simulink model "soft_finger_main"  (R2022b)
settings: Solver=VariableStepAuto  StartTime=0.0  StopTime=50  RelTol=1e-3
undefined symbols (not defined in the file): bounds, cf, D, DiscIntNeverNeededParam, Discrete, Fingertip, forceSetPoint, K, M, mylib, rho, sensor_locs, Time, X, Y, Z
libraries: sm_lib x117, nesl_utility x97, fl_lib x81, ee_lib x6, simulink x4, statsLibrary x3, slpidlib x2, deeplib x1, ctrlSharedLib x1
(part 1 of 5)
settings Model: Creator=toby  LastModifiedBy=chapa
settings SolverCC: AlgebraicLoopSolver=TrustRegion
settings DebuggingCC: UnconnectedInputMsg=warning  UnconnectedOutputMsg=warning  UnconnectedLineMsg=warning  SFMachineParentedDataDiag=warning
settings ModelReferenceCC: EnableRefExpFcnMdlSchedulingChecks=on
settings RTWCC: DLArmComputeVersion=19.05
settings ExplorerConfigSet: InternalSimMechanicsExplorerSettings="<ExplorerConfiguration><canonicalview>default</canonicalview><AnimationSetting><BasePlaybackSpeed>1.0</BasePlaybackSpeed><PlaybackSpeedFactor>1.0</PlaybackSpeedFactor></AnimationSetting><TilePanel><TileInfo><Tiles Columns=\"1\" Count=\"1\" Rows=\"1\"><Column Weight=\"1\"/><Row Weight=\"1\"/><Tile Height=\"1\" Width=\"1\" X=\"0\" Y=\"0\"/></Tiles></TileInfo><SceneInfo><SceneViewer><BGColor><R>1</R><G>1</G><B>1</B></BGColor><Camera><DoPerspective>off</DoPerspective><Position><X>0.648695100589207763</X><Y>-0.590632325015253423</Y><Z>0.584680131044784668</Z></Position><Center><X>0.0713448313995819899</X><Y>-0.0132820558256276505</Y><Z>0.0073298618551588552</Z></Center><Up><X>-0.408248290463863073</X><Y>0.408248290463863073</Y><Z>0.816496580927726145</Z></Up><ViewLimDist>1</ViewLimDist><YLim>0.069189024666258106</YLim><XLim>0.106148631121814288</XLim></Camera></SceneViewer></SceneInfo></TilePanel><MechEditorPanel><Cameras/><GfxPanelCameraMap/><VideoCreator><PlaybackSpeedRatio>1.0</PlaybackSpeedRatio><FrameRate>30</FrameRate><VideoFormat>Motion JPEG AVI</VideoFormat><FrameSize>auto</FrameSize></VideoCreator></MechEditorPanel></ExplorerConfiguration>"

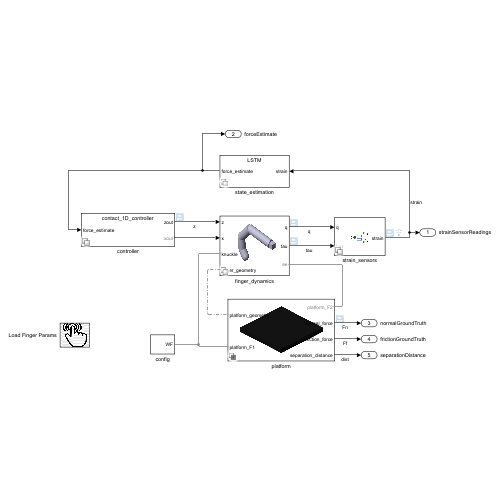
[thumbnail: Simulink's stored preview of the top-level diagram]
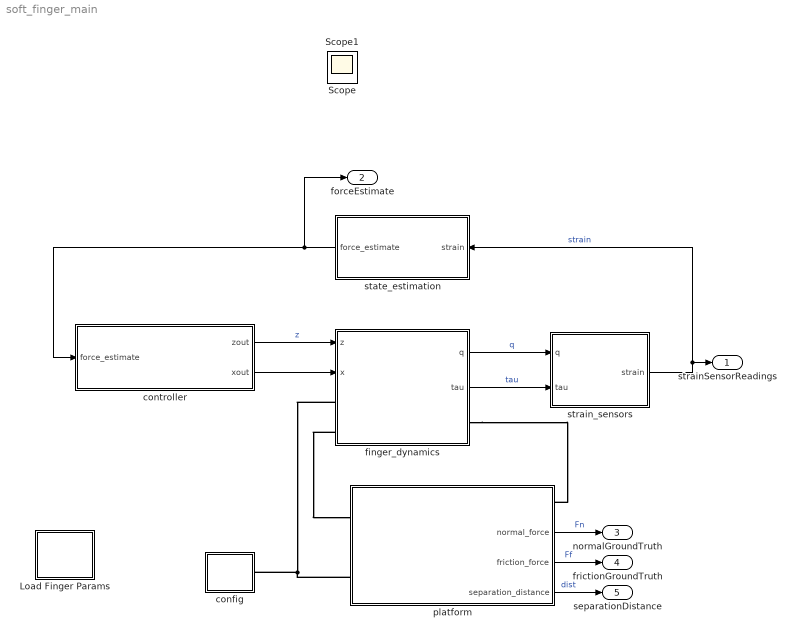
== system soft_finger_main ==
  Load Finger Params : Subsystem
      settings: OpenFcn=loadFingerParams;
      mask Display: image('$imagefile'); % Use "Edit Image" on toolstrip to change.
  config : Subsystem
  controller : Subsystem  Variant=on  VariantControl=Choice
  finger_dynamics : Subsystem  Variant=on  VariantControl=Choice
      mask Display: image('$imagefile'); % Use "Edit Image" on toolstrip to change.
  platform : Subsystem  Variant=on  VariantControlMode=label  VariantControl=Choice  LabelModeActiveChoice=long_2D
      settings: PortSchema="{\"entries\":[{\"content\":{\"sides\":[{\"content\":{\"connectorIds\":[\"LConn1\",\"LConn2\"]},\"type\":\"ConnectorPlacement.EquallySpacedRectSide\",\"uuid\":\"48745db0-03fd-4998-bcf1-1a9aed8c42d1\"},{\"content\":{\"connectorIds\":[\"RConn1\",\"Out1\",\"Out2\",\"Out3\"],\"side\":\"RIGHT\"},\"type\":\"ConnectorPlacement.EquallySpacedRectSide\",\"uuid\":\"a3eff733-8e96-4ac6-b0c1-c9eca8eafbf9\"},{\"content\":{\"connectorIds\":[],\"side\":\"TOP\"},\"type\":\"ConnectorPlacement.EquallySpacedRectSide\",\"uuid\":\"624833be-01c7-4c79-8903-c72d4883aa5d\"}]},\"type\":\"ConnectorPlacement.EquallySpacedConnector\",\"uuid\":\"3e612e1c-fe4d-4d00-a236-ee36b2ab6a58\"}],\"packageUris\":[\"http://schema.mathworks.com/mf0/Connector/R2020b\"],\"version\":\"1.0\"}"
      mask Display: image('$imagefile'); % Use "Edit Image" on toolstrip to change.
  state_estimation : Subsystem  Variant=on  VariantControl=Choice
  strain_sensors : Subsystem  Variant=on  VariantControl=Choice
      mask Display: image('$imagefile'); % Use "Edit Image" on toolstrip to change.
  strainSensorReadings : Outport
  forceEstimate : Outport  Port=2
  normalGroundTruth : Outport  Port=3
  frictionGroundTruth : Outport  Port=4
  separationDistance : Outport  Port=5
  Scope : Scope
  Scope1 : Scope
  wires:
  strain_sensors/1(strain) -> state_estimation/1(strain), strainSensorReadings/1  "strain"
  platform/1(normal_force) -> normalGroundTruth/1  "Fn"
  controller/1(zout) -> finger_dynamics/1(z)  "z"
  finger_dynamics/1(q) -> strain_sensors/1(q)  "q"
  state_estimation/1(force_estimate) -> controller/1(force_estimate), forceEstimate/1
  controller/2(xout) -> finger_dynamics/2(x)
  platform/2(friction_force) -> frictionGroundTruth/1  "Ff"
  platform/3(separation_distance) -> separationDistance/1  "dist"
  finger_dynamics/2(tau) -> strain_sensors/2(tau)  "tau"
  connections:
  platform/LConn2 -- config/RConn1 -- finger_dynamics/LConn1
  finger_dynamics/LConn2 -- platform/LConn1
  finger_dynamics/RConn1 -- platform/RConn1

== system soft_finger_main/Load Finger Params ==

== system soft_finger_main/config ==
  Mechanism Configuration : sm_lib/Utilities/Mechanism Configuration  UniformGravity=Constant  GravityVector=[0 0 -9.80665]  GravityUnits=m/s^2  LinearizationDelta=0.001  JointModeTransitionNonlinearIterations=2
  Solver Configuration : nesl_utility/Solver Configuration  PhysicalDomain=network_engine_domain  SubClassName=solver  LeftPortType=input  RightPortType=generic  Tones=[]  Harmonics=[]  SimulateNoise=off  Profile=off  UseLocalSampling=off  EnableSwitchedLinearOptims=on  FrequencyDomain=off  UseCCode=off  RelTol=0.001  AbsTol=1e-06  MinStep=1e-09  ToWorkspace=off  RevertToSquareIcSolve=off  NumHomotopyIterations=100  PhasorMode=off  PhasorModeNumHarmonics=1  ConsistencySolver=NEWTON_XTOL_AFTER_FTOL  IndexReductionMethod=DerivativeReplacement  DoDC=off  ResidualTolerance=1e-09  ConsistencyTolSource=GLOBAL  ConsistencyAbsTol=0.001  ConsistencyRelTol=0.001  ConsistencyTolFactor=0.001  UseLocalSolver=off  LocalSolverChoice=NE_BACKWARD_EULER_ADVANCER  ResolveIndetEquations=on  FunctionEvalNumThread=1  LocalSolverSampleTime=0.001  DoFixedCost=off  MaxNonlinIter=3  MaxModeIter=2  ComputeImpulses=off  ImpulseIterations=2  LinearAlgebra=auto  LinearAlgebraNumThread=0  EquationFormulation=NE_TIME_EF  DelaysMemoryBudget=1024  AutomaticFiltering=on  FilteringTimeConstant=0.001  PartitionStorageMethod=AS_NEEDED  PartitionMemoryBudget=1024  PartitionMethod=ROBUST
  World Frame : sm_lib/Frames and Transforms/World Frame
  WF : PMIOPort  Side=Right
  connections:
  Mechanism Configuration/RConn1 -- WF/RConn1 -- World Frame/RConn1 -- Solver Configuration/RConn1

== system soft_finger_main/controller ==
  force_estimate : Inport
  contact_1D_controller : Subsystem  VariantControl=controller_choice==1
  contact_2D_controller : Subsystem  VariantControl=controller_choice==2
  custom : Subsystem  VariantControl=controller_choice==2
  random_walker_xz : Subsystem  VariantControl=controller_choice==4
  random_walker_z : Subsystem  VariantControl=controller_choice==3
  zout : Outport
  xout : Outport  Port=2

== system soft_finger_main/finger_dynamics ==
  z : Inport
  x : Inport  Port=2
  XZ Translation at Base : Subsystem  VariantControl=plant_choice == 2
  Z Translation at Base : Subsystem  VariantControl=plant_choice == 1
  knuckle : PMIOPort  Side=Left
  finger_geometry : PMIOPort  Port=2  Side=Left
  ee : PMIOPort  Port=3  Side=Right
  q : Outport
  tau : Outport  Port=2

== system soft_finger_main/platform ==
  long_platform : Subsystem  VariantControl=long_2D
  short_platform : Subsystem  VariantControl=short_1D
  platform_geometry : PMIOPort  Side=Left
  platform_F1 : PMIOPort  Port=2  Side=Left
  platform_F2 : PMIOPort  Port=3  Side=Right
  normal_force : Outport
  friction_force : Outport  Port=2
  separation_distance : Outport  Port=3

== system soft_finger_main/state_estimation ==
  strain : Inport
  LSTM : Subsystem  VariantControl=observer_choice == 3
      settings: AttributesFormatString=(Experimental)
  SVM : Subsystem  VariantControl=observer_choice == 4
  bagged_ensemble : Subsystem  VariantControl=observer_choice == 1
  bagged_ensemble_with_friction : Subsystem  VariantControl=observer_choice == 2
  custom : Subsystem  VariantControl=observer_choice == 8
  kalman_filter : Subsystem  VariantControl=observer_choice == 7
      settings: AttributesFormatString=(Experimental)
  linear_regression : Subsystem  VariantControl=observer_choice == 5
  off : Subsystem  VariantControl=observer_choice == 9
  state_space_observer : Subsystem  VariantControl=observer_choice == 6
      settings: AttributesFormatString=(Experimental)
  force_estimate : Outport

== system soft_finger_main/strain_sensors ==
  q : Inport
  tau : Inport  Port=2
  drifting_strain_sensor : Subsystem  VariantControl=sensor_choice == 1
  ssc_strain_sensor : Subsystem  VariantControl=sensor_choice == 2
  strain : Outport

== system soft_finger_main/controller/contact_1D_controller ==
  note: adjust the force set point and observe at which force the mechanism collapses
  force_estimate : Inport
  Bus Selector : BusSelector  OutputSignals=normal
  Delay2 : Delay  DelayLength=1;  InitialCondition=0;
  PID Controller : slpidlib/PID Controller  Controller=PID  Form=Parallel  TimeDomain=Discrete-time  UseExternalTs=off  SampleTime=-1  IntegratorMethod=Forward Euler  FilterMethod=Forward Euler  ControllerParametersSource=internal  P=1.4  I=0  UseKiTs=off  D=0.05  N=1  UseFilter=on  TunerSelectOption=Frequency Response Based  InitialConditionSource=internal  InitialConditionForIntegrator=0  InitialConditionForFilter=0  DifferentiatorICPrevScaledInput=0  ExternalReset=none  TrackingMode=off  Kt=1  LimitOutput=off  SatLimitsSource=internal  UpperSaturationLimit=inf  LowerSaturationLimit=-inf  LinearizeAsGain=on  AntiWindupMode=none  Kb=1  LimitIntegrator=off  UpperIntegratorSaturationLimit=inf  LowerIntegratorSaturationLimit=-inf  POutMin=[]  POutMax=[]  IOutMin=[]  IOutMax=[]  DOutMin=[]  DOutMax=[]  NOutMin=[]  NOutMax=[]  SumOutMin=[]  SumOutMax=[]  SaturationOutMin=[]  SaturationOutMax=[]  PParamMin=[]  PParamMax=[]  IParamMin=[]  IParamMax=[]  DParamMin=[]  DParamMax=[]  NParamMin=[]  NParamMax=[]  KbParamMin=[]  KbParamMax=[]  KtParamMin=[]  KtParamMax=[]  KbOutMin=[]  KbOutMax=[]  KtOutMin=[]  KtOutMax=[]  IntegratorOutMin=[]  IntegratorOutMax=[]  FilterOutMin=[]  FilterOutMax=[]  SumI1OutMin=[]  SumI1OutMax=[]  SumI2OutMin=[]  SumI2OutMax=[]  SumI3OutMin=[]  SumI3OutMax=[]  SumI4OutMin=[]  SumI4OutMax=[]  SumDOutMin=[]  SumDOutMax=[]  DifferentiatorOutMin=[]  DifferentiatorOutMax=[]  FilterDiffOutCoefMin=[]  FilterDiffOutCoefMax=[]  ReciprocalOutMin=[]  ReciprocalOutMax=[]  SumDenOutMin=[]  SumDenOutMax=[]  SumNumOutMin=[]  SumNumOutMax=[]  DivideOutMin=[]  DivideOutMax=[]  UdiffTsProdOutMin=[]  UdiffTsProdOutMax=[]  NTsProdOutMin=[]  NTsProdOutMax=[]  UintegralTsProdOutMin=[]  UintegralTsProdOutMax=[]  UngainTsProdOutMin=[]  UngainTsProdOutMax=[]  ClampingZeroOutDataTypeStr=Inherit: Inherit via back propagation  ClampingZeroOutMin=[]  ClampingZeroOutMax=[]  FilterDenConstantOutDataTypeStr=Inherit: Inherit via back propagation  FilterDenConstantOutMin=[]  FilterDenConstantOutMax=[]  PCopyOutDataTypeStr=Inherit: Inherit via back propagation  PCopyOutMin=[]  PCopyOutMax=[]  NCopyOutDataTypeStr=Inherit: Inherit via back propagation  NCopyOutMin=[]  NCopyOutMax=[]  IntegratorContinuousStateAttributes=''  IntegratorStateMustResolveToSignalObject=off  IntegratorRTWStateStorageClass=Auto  FilterContinuousStateAttributes=''  FilterStateMustResolveToSignalObject=off  FilterRTWStateStorageClass=Auto  ParallelPVariant=InternalParameters  IdealPVariant=Disabled  IVariant=InternalParameters  DVariant=InternalParameters  IntegratorVariant=Discrete  SatVariant=Disabled  AWVariant=Passthrough  PCopyVariant=Disabled  TRVariant=Disabled  FdbkBlocksVariant=Forward  IdealPFdbkVariant=Disabled  SatFdbkVariant=Disabled  DerivativeFilterVariant=ForwardEulerFilter  NVariant=InternalParameters  NCopyVariant=Disabled  FilterICVariant=InternalICsFilter  IntegratorICVariant=InternalICs  ExternalResetVariant=Disabled  TRSumVariant=Passthrough  SumFdbkVariant=Disabled  SumVariant=Sum_PID  TsampFilterVariant=InternalTs  TsampNgainVariant=Passthrough  TsampIntegralVariant=Passthrough  ExternalSaturationOutDataTypeStr=Inherit: Same as second input
  Sum1 : Sum  Inputs=|+-
  Sum2 : Sum  Inputs=|-+
  Zero-Order Hold : ZeroOrderHold  SampleTime=-1
  acceleration limiter : Subsystem
  desired_force : Constant  Value=forceSetPoint
  zout : Outport
  wires:
  force_estimate/1 -> Bus Selector/1
  Sum1/1 -> PID Controller/1  "forceErr"
  acceleration limiter/1(zout) -> zout/1
  Sum2/1 -> Zero-Order Hold/1, Delay2/1  "pos_next"
  Delay2/1 -> Sum2/2  "pos_now"
  Zero-Order Hold/1 -> acceleration limiter/1(pos_next)
  PID Controller/1 -> Sum2/1  "pos_fb_correction"
  desired_force/1 -> Sum1/1  "sp"
  Bus Selector/1 -> Sum1/2  "<normal>"

== system soft_finger_main/controller/contact_2D_controller ==
  note: adjust the force set point and observe at which force the mechanism collapses
  force_estimate : Inport
  Bus Selector : BusSelector  OutputSignals=normal
  Bus Selector1 : BusSelector  OutputSignals=friction
  Delay2 : Delay  DelayLength=1;  InitialCondition=0;
  PID Controller : slpidlib/PID Controller  Controller=PID  Form=Parallel  TimeDomain=Discrete-time  UseExternalTs=off  SampleTime=-1  IntegratorMethod=Forward Euler  FilterMethod=Forward Euler  ControllerParametersSource=internal  P=1.4  I=0  UseKiTs=off  D=0.05  N=1  UseFilter=on  TunerSelectOption=Frequency Response Based  InitialConditionSource=internal  InitialConditionForIntegrator=0  InitialConditionForFilter=0  DifferentiatorICPrevScaledInput=0  ExternalReset=none  TrackingMode=off  Kt=1  LimitOutput=off  SatLimitsSource=internal  UpperSaturationLimit=inf  LowerSaturationLimit=-inf  LinearizeAsGain=on  AntiWindupMode=none  Kb=1  LimitIntegrator=off  UpperIntegratorSaturationLimit=inf  LowerIntegratorSaturationLimit=-inf  POutMin=[]  POutMax=[]  IOutMin=[]  IOutMax=[]  DOutMin=[]  DOutMax=[]  NOutMin=[]  NOutMax=[]  SumOutMin=[]  SumOutMax=[]  SaturationOutMin=[]  SaturationOutMax=[]  PParamMin=[]  PParamMax=[]  IParamMin=[]  IParamMax=[]  DParamMin=[]  DParamMax=[]  NParamMin=[]  NParamMax=[]  KbParamMin=[]  KbParamMax=[]  KtParamMin=[]  KtParamMax=[]  KbOutMin=[]  KbOutMax=[]  KtOutMin=[]  KtOutMax=[]  IntegratorOutMin=[]  IntegratorOutMax=[]  FilterOutMin=[]  FilterOutMax=[]  SumI1OutMin=[]  SumI1OutMax=[]  SumI2OutMin=[]  SumI2OutMax=[]  SumI3OutMin=[]  SumI3OutMax=[]  SumI4OutMin=[]  SumI4OutMax=[]  SumDOutMin=[]  SumDOutMax=[]  DifferentiatorOutMin=[]  DifferentiatorOutMax=[]  FilterDiffOutCoefMin=[]  FilterDiffOutCoefMax=[]  ReciprocalOutMin=[]  ReciprocalOutMax=[]  SumDenOutMin=[]  SumDenOutMax=[]  SumNumOutMin=[]  SumNumOutMax=[]  DivideOutMin=[]  DivideOutMax=[]  UdiffTsProdOutMin=[]  UdiffTsProdOutMax=[]  NTsProdOutMin=[]  NTsProdOutMax=[]  UintegralTsProdOutMin=[]  UintegralTsProdOutMax=[]  UngainTsProdOutMin=[]  UngainTsProdOutMax=[]  ClampingZeroOutDataTypeStr=Inherit: Inherit via back propagation  ClampingZeroOutMin=[]  ClampingZeroOutMax=[]  FilterDenConstantOutDataTypeStr=Inherit: Inherit via back propagation  FilterDenConstantOutMin=[]  FilterDenConstantOutMax=[]  PCopyOutDataTypeStr=Inherit: Inherit via back propagation  PCopyOutMin=[]  PCopyOutMax=[]  NCopyOutDataTypeStr=Inherit: Inherit via back propagation  NCopyOutMin=[]  NCopyOutMax=[]  IntegratorContinuousStateAttributes=''  IntegratorStateMustResolveToSignalObject=off  IntegratorRTWStateStorageClass=Auto  FilterContinuousStateAttributes=''  FilterStateMustResolveToSignalObject=off  FilterRTWStateStorageClass=Auto  ParallelPVariant=InternalParameters  IdealPVariant=Disabled  IVariant=InternalParameters  DVariant=InternalParameters  IntegratorVariant=Discrete  SatVariant=Disabled  AWVariant=Passthrough  PCopyVariant=Disabled  TRVariant=Disabled  FdbkBlocksVariant=Forward  IdealPFdbkVariant=Disabled  SatFdbkVariant=Disabled  DerivativeFilterVariant=ForwardEulerFilter  NVariant=InternalParameters  NCopyVariant=Disabled  FilterICVariant=InternalICsFilter  IntegratorICVariant=InternalICs  ExternalResetVariant=Disabled  TRSumVariant=Passthrough  SumFdbkVariant=Disabled  SumVariant=Sum_PID  TsampFilterVariant=InternalTs  TsampNgainVariant=Passthrough  TsampIntegralVariant=Passthrough  ExternalSaturationOutDataTypeStr=Inherit: Same as second input
  Sine Wave : Sin  Amplitude=5  Frequency=0.5  SampleTime=0
  Sum1 : Sum  Inputs=|+-
  Sum2 : Sum  Inputs=|-+
  Terminator : Terminator
  Zero-Order Hold : ZeroOrderHold  SampleTime=-1
  acceleration limiter : Subsystem
  desired_force : Constant  Value=0.1
  zout : Outport
  xout : Outport  Port=2
  wires:
  PID Controller/1 -> Sum2/1  "pos_fb_correction"
  Zero-Order Hold/1 -> acceleration limiter/1(pos_next)
  Delay2/1 -> Sum2/2  "pos_now"
  Sum2/1 -> Delay2/1, Zero-Order Hold/1  "pos_next"
  acceleration limiter/1(zout) -> zout/1
  Sum1/1 -> PID Controller/1  "forceErr"
  Sine Wave/1 -> xout/1  "xref"
  desired_force/1 -> Sum1/1  "sp"
  force_estimate/1 -> Bus Selector1/1, Bus Selector/1
  Bus Selector/1 -> Sum1/2  "<normal>"
  Bus Selector1/1 -> Terminator/1  "<friction>"

== system soft_finger_main/controller/custom ==
  force_estimate : Inport
  Bus Selector : BusSelector  OutputSignals=normal
  Bus Selector1 : BusSelector  OutputSignals=friction
  Constant : Constant  Value=0
  Constant1 : Constant  Value=0
  Terminator : Terminator
  Terminator1 : Terminator
  zout : Outport
  xout : Outport  Port=2
  wires:
  Bus Selector1/1 -> Terminator/1  "<friction>"
  force_estimate/1 -> Bus Selector/1, Bus Selector1/1
  Bus Selector/1 -> Terminator1/1  "<normal>"
  Constant/1 -> zout/1
  Constant1/1 -> xout/1

== system soft_finger_main/controller/random_walker_xz ==
  Add1 : Sum  Inputs=+-+
  Add2 : Sum  Inputs=+-+
  Saturation : Saturate  UpperLimit=bounds(1)  LowerLimit=bounds(2)
  Saturation1 : Saturate  UpperLimit=10  LowerLimit=-10
  Sum : Sum  Inputs=-+|
  Sum1 : Sum  Inputs=-+|
  Unit Delay{1..4} (4 alike) : UnitDelay  SampleTime=-1  HasFrameUpgradeWarning=on
  random dx : RandomNumber  Variance=10  SampleTime=0.1
  random dz : RandomNumber  Variance=0.1  Seed=1  SampleTime=0.1
  zout : Outport
  xout : Outport  Port=2
  wires:
  Unit Delay1/1 -> Add1/3  "ztminus1"
  random dz/1 -> Add1/1
  Add1/1 -> Sum/2, Saturation/1, Unit Delay1/1  "zt"
  Sum/1 -> Unit Delay3/1  "anitwindupz"
  Saturation/1 -> Sum/1, zout/1  "zout"
  Saturation1/1 -> xout/1, Sum1/1  "xout"
  Sum1/1 -> Unit Delay4/1  "anitwindupx"
  Add2/1 -> Saturation1/1, Sum1/2, Unit Delay2/1  "xt"
  random dx/1 -> Add2/1
  Unit Delay2/1 -> Add2/3  "xtminus1"
  Unit Delay3/1 -> Add1/2  "ztminus1"
  Unit Delay4/1 -> Add2/2  "ztminus1"

== system soft_finger_main/controller/random_walker_z ==
  Add1 : Sum  Inputs=+-+
  Constant6 : Constant  Commented=on  Value=[bounds]
  Constant7 : Constant  Commented=on  Value=cf
  Delay : Delay  Commented=on  DelayLength=1;  InitialCondition=[10, 0, 1, 1, 1];
  Demux : Demux  Commented=on  Outputs=5
  MATLAB Function2 : MATLAB Function  Commented=on  TreatAsAtomicUnit=on
  Mux1 : Mux  Commented=on  Inputs=5
  Rate Transition : RateTransition  Commented=on  InitialCondition=0;  OutPortSampleTime=1/cf;
  Saturation : Saturate  UpperLimit=bounds(1)  LowerLimit=bounds(2)
  Sum : Sum  Inputs=-+|
  Unit Delay1 : UnitDelay  SampleTime=-1  HasFrameUpgradeWarning=on
  Unit Delay2 : UnitDelay  SampleTime=-1  HasFrameUpgradeWarning=on
  acceleration limiter : Subsystem  Commented=on
  random dz : RandomNumber  Variance=0.1  Seed=1  SampleTime=0.1
  zout : Outport
  wires:
  Delay/1 -> Demux/1
  Demux/5 -> MATLAB Function2/5("step_no ")
  Demux/1 -> MATLAB Function2/1(pos_now)
  MATLAB Function2/2(pos_goal) -> Mux1/2
  Demux/3 -> MATLAB Function2/3("thres ")
  MATLAB Function2/5(step_no) -> Mux1/5
  Demux/4 -> MATLAB Function2/4("batch ")
  Demux/2 -> MATLAB Function2/2("pos_goal ")
  MATLAB Function2/4(batch) -> Mux1/4
  Rate Transition/1 -> Delay/1
  Mux1/1 -> Rate Transition/1
  MATLAB Function2/1(pos_next) -> Mux1/1, acceleration limiter/1(pos_next)
  Constant7/1 -> MATLAB Function2/7(cf)
  Constant6/1 -> MATLAB Function2/6(bounds)
  MATLAB Function2/3(thres) -> Mux1/3
  acceleration limiter/1(zout) -> ?
  Sum/1 -> Unit Delay2/1  "anitwindupz"
  random dz/1 -> Add1/1
  Unit Delay1/1 -> Add1/3  "ztminus1"
  Saturation/1 -> zout/1, Sum/1  "zout"
  Add1/1 -> Sum/2, Saturation/1, Unit Delay1/1  "zt"
  Unit Delay2/1 -> Add1/2  "ztminus1"

== system soft_finger_main/finger_dynamics/XZ Translation at Base ==
  z : Inport
  x : Inport  Port=2
  Terminator : Terminator
  finger : Subsystem
      mask Display: image('$imagefile'); % Use "Edit Image" on toolstrip to change.
  knuckle : PMIOPort  Side=Left
  finger_geometry : PMIOPort  Port=2  Side=Left
  ee : PMIOPort  Port=3  Side=Right
  q : Outport
  tau : Outport  Port=2
  wires:
  finger/1(joint_angles) -> q/1  "q"
  z/1 -> finger/1(z)
  x/1 -> finger/2(x)
  finger/3(joint_torques) -> tau/1
  finger/2(joint_forces) -> Terminator/1
  connections:
  knuckle/RConn1 -- finger/LConn1
  finger/LConn2 -- finger_geometry/RConn1
  finger/RConn1 -- ee/RConn1

== system soft_finger_main/finger_dynamics/Z Translation at Base ==
  z : Inport
  Terminator : Terminator
  finger : Subsystem
      mask Display: image('$imagefile'); % Use "Edit Image" on toolstrip to change.
  knuckle : PMIOPort  Side=Left
  finger_geometry : PMIOPort  Port=2  Side=Left
  ee : PMIOPort  Port=3  Side=Right
  q : Outport
  tau : Outport  Port=2
  wires:
  z/1 -> finger/1(z)
  finger/1(joint_angles) -> q/1  "q"
  finger/3(joint_torques) -> tau/1  "tau"
  finger/2(joint_forces) -> Terminator/1
  connections:
  ee/RConn1 -- finger/RConn1
  finger_geometry/RConn1 -- finger/LConn2
  knuckle/RConn1 -- finger/LConn1

== system soft_finger_main/platform/long_platform ==
  platform : Subsystem
      settings: PortSchema="{\"entries\":[{\"content\":{\"sides\":[{\"content\":{\"connectorIds\":[\"LConn1\",\"LConn2\"]},\"type\":\"ConnectorPlacement.EquallySpacedRectSide\",\"uuid\":\"6339b0d2-d5db-4d9b-bf7c-b55391eb7ced\"},{\"content\":{\"connectorIds\":[\"RConn1\",\"Out1\",\"Out2\",\"Out3\"],\"side\":\"RIGHT\"},\"type\":\"ConnectorPlacement.EquallySpacedRectSide\",\"uuid\":\"c0a265d5-31ed-4e5e-b9ed-737d24bd79ad\"},{\"content\":{\"connectorIds\":[],\"side\":\"TOP\"},\"type\":\"ConnectorPlacement.EquallySpacedRectSide\",\"uuid\":\"95fda260-2475-4278-80fa-e6b57f61896e\"}]},\"type\":\"ConnectorPlacement.EquallySpacedConnector\",\"uuid\":\"d01ea818-4985-47a8-ad3c-f52aaf4b2cf0\"}],\"packageUris\":[\"http://schema.mathworks.com/mf0/Connector/R2020b\"],\"version\":\"1.0\"}"
      mask Display: image('$imagefile'); % Use "Edit Image" on toolstrip to change.
  platform_geometry : PMIOPort  Side=Left
  platform_F1 : PMIOPort  Port=2  Side=Left
  platform_F2 : PMIOPort  Port=3  Side=Right
  normal_force : Outport
  friction_force : Outport  Port=2
  separation_distance : Outport  Port=3
  wires:
  platform/1(normal_force) -> normal_force/1  "nfgt"
  platform/2(friction_force) -> friction_force/1  "ffgt"
  platform/3(separation_distance) -> separation_distance/1  "dist"
  connections:
  platform/LConn2 -- platform_F1/RConn1
  platform/RConn1 -- platform_F2/RConn1
  platform/LConn1 -- platform_geometry/RConn1

== system soft_finger_main/platform/short_platform ==
  platform : Subsystem
      settings: PortSchema="{\"entries\":[{\"content\":{\"sides\":[{\"content\":{\"connectorIds\":[\"LConn1\",\"LConn2\"]},\"type\":\"ConnectorPlacement.EquallySpacedRectSide\",\"uuid\":\"6339b0d2-d5db-4d9b-bf7c-b55391eb7ced\"},{\"content\":{\"connectorIds\":[\"RConn1\",\"Out1\"],\"side\":\"RIGHT\"},\"type\":\"ConnectorPlacement.EquallySpacedRectSide\",\"uuid\":\"c0a265d5-31ed-4e5e-b9ed-737d24bd79ad\"},{\"content\":{\"connectorIds\":[],\"side\":\"TOP\"},\"type\":\"ConnectorPlacement.EquallySpacedRectSide\",\"uuid\":\"95fda260-2475-4278-80fa-e6b57f61896e\"}]},\"type\":\"ConnectorPlacement.EquallySpacedConnector\",\"uuid\":\"d01ea818-4985-47a8-ad3c-f52aaf4b2cf0\"}],\"packageUris\":[\"http://schema.mathworks.com/mf0/Connector/R2020b\"],\"version\":\"1.0\"}"
      mask Display: image('$imagefile'); % Use "Edit Image" on toolstrip to change.
  platform_geometry : PMIOPort  Side=Left
  platform_F1 : PMIOPort  Port=2  Side=Left
  platform_F2 : PMIOPort  Port=3  Side=Right
  normal_force : Outport
  wires:
  platform/1(normal_force) -> normal_force/1
  connections:
  platform/LConn1 -- platform_geometry/RConn1
  platform/RConn1 -- platform_F2/RConn1
  platform_F1/RConn1 -- platform/LConn2

== system soft_finger_main/state_estimation/LSTM ==
  strain : Inport
  Bus Creator : BusCreator  Inputs=1
  Rate Transition : RateTransition  InitialCondition=0;  OutPortSampleTime=1/cf;
  Stateful Predict : deeplib/Stateful Predict  Network=Network from MAT-file  NetworkFunction=untitled  NetworkFilePath=ml_models\lstm2.mat  InputDataFormats={ '', '' }  SampleTime=0.04  ForceInterpretedSim=off  EnableDLNetwork=on
  Unit Delay : UnitDelay  SampleTime=-1  HasFrameUpgradeWarning=on
  force_estimate : Outport
  wires:
  strain/1 -> Unit Delay/1
  Stateful Predict/1 -> Rate Transition/1
  Unit Delay/1 -> Stateful Predict/1
  Rate Transition/1 -> Bus Creator/1  "normal"
  Bus Creator/1 -> force_estimate/1

== system soft_finger_main/state_estimation/SVM ==
  strain : Inport
  Bus Creator : BusCreator  Inputs=1
  MATLAB Function : MATLAB Function  TreatAsAtomicUnit=on
  Rate Transition : RateTransition  InitialCondition=0;  OutPortSampleTime=1/cf;
  Transpose : Math  Operator=transpose
  Unit Delay : UnitDelay  SampleTime=-1  HasFrameUpgradeWarning=on
  force_estimate : Outport
  wires:
  Unit Delay/1 -> Transpose/1
  MATLAB Function/1(force) -> Rate Transition/1
  strain/1 -> Unit Delay/1
  Transpose/1 -> MATLAB Function/1(Strain)
  Rate Transition/1 -> Bus Creator/1  "normal"
  Bus Creator/1 -> force_estimate/1

== system soft_finger_main/state_estimation/bagged_ensemble ==
  strain : Inport
  Bus Creator : BusCreator  Inputs=1
  Rate Transition : RateTransition  InitialCondition=0;  OutPortSampleTime=1/cf;
  Unit Delay : UnitDelay  SampleTime=-1  HasFrameUpgradeWarning=on
  bagged ensemble state estimator : statsLibrary/Regression/RegressionEnsemble Predict  TrainedLearner=ensMdl  OutMin=[]  OutMax=[]  WeakLearnerOutMin=[]  WeakLearnerOutMax=[]
  force_estimate : Outport
  wires:
  Unit Delay/1 -> bagged ensemble state estimator/1
  bagged ensemble state estimator/1 -> Rate Transition/1
  strain/1 -> Unit Delay/1
  Rate Transition/1 -> Bus Creator/1  "normal"
  Bus Creator/1 -> force_estimate/1

== system soft_finger_main/state_estimation/bagged_ensemble_with_friction ==
  strain : Inport
  Bus Creator : BusCreator  Inputs=2
  Rate Transition : RateTransition  InitialCondition=0;  OutPortSampleTime=1/cf;
  Rate Transition1 : RateTransition  InitialCondition=0;  OutPortSampleTime=1/cf;
  Unit Delay : UnitDelay  SampleTime=-1  HasFrameUpgradeWarning=on
  Unit Delay1 : UnitDelay  SampleTime=-1  HasFrameUpgradeWarning=on
  "bagged ensemble friction state estimator " : statsLibrary/Regression/RegressionEnsemble Predict  TrainedLearner=frictionForceModel  OutMin=[]  OutMax=[]  WeakLearnerOutMin=[]  WeakLearnerOutMax=[]
  bagged ensemble normal state estimator : statsLibrary/Regression/RegressionEnsemble Predict  TrainedLearner=normalForceModel  OutMin=[]  OutMax=[]  WeakLearnerOutMin=[]  WeakLearnerOutMax=[]
  force_estimate : Outport
  wires:
  Bus Creator/1 -> force_estimate/1
  Rate Transition/1 -> Bus Creator/1  "normal"
  strain/1 -> Unit Delay1/1, Unit Delay/1
  bagged ensemble normal state estimator/1 -> Rate Transition/1
  Unit Delay/1 -> bagged ensemble normal state estimator/1
  Unit Delay1/1 -> "bagged ensemble friction state estimator "/1
  "bagged ensemble friction state estimator "/1 -> Rate Transition1/1
  Rate Transition1/1 -> Bus Creator/2  "friction"

== system soft_finger_main/state_estimation/custom ==
  strain : Inport
  Bus Creator : BusCreator  Inputs=2
  Rate Transition : RateTransition  InitialCondition=0;  OutPortSampleTime=1/cf;
  Rate Transition1 : RateTransition  InitialCondition=0;  OutPortSampleTime=1/cf;
  Unit Delay : UnitDelay  SampleTime=-1  HasFrameUpgradeWarning=on
  Unit Delay1 : UnitDelay  SampleTime=-1  HasFrameUpgradeWarning=on
  friction_state_estimator : Subsystem
  normal_force_state_estimator : Subsystem
  force_estimate : Outport
  wires:
  Rate Transition1/1 -> Bus Creator/2  "friction"
  friction_state_estimator/1(Out1) -> Rate Transition1/1
  Unit Delay1/1 -> friction_state_estimator/1(In1)
  Unit Delay/1 -> normal_force_state_estimator/1(In1)
  normal_force_state_estimator/1(Out1) -> Rate Transition/1
  strain/1 -> Unit Delay/1, Unit Delay1/1
  Rate Transition/1 -> Bus Creator/1  "normal"
  Bus Creator/1 -> force_estimate/1

== system soft_finger_main/state_estimation/kalman_filter ==
  strain : Inport
  Bus Creator : BusCreator  Inputs=1
  Rate Transition : RateTransition  InitialCondition=0;  OutPortSampleTime=1/cf;
  SysID Kalman Filter : ctrlSharedLib/Kalman Filter  TimeDomain=Discrete-Time  UseCurrentEstimator=on  ModelSource=LTI State-Space Variable  ModelSourceVariable=ss(0.95,1,1,0,1)  A=0.95  B=1  C=1  D=0  NumberOfStates=1  NumberOfInputs=1  NumberOfOutputs=1  InitialEstimateSource=Dialog  X0=0  P0=10  UseK=off  UseGH=off  NumberOfProcessNoiseInputs=1  G=1  TimeInvariantG=on  H=0  TimeInvariantH=on  Q=0.05  TimeInvariantQ=on  R=1  TimeInvariantR=on  N=0  TimeInvariantN=on  AddInputPort=off  AddEnablePort=off  OutputEstimatedY=off  OutputP=off  Ts=-1
  Unit Delay : UnitDelay  SampleTime=-1  HasFrameUpgradeWarning=on
  force_estimate : Outport
  wires:
  Unit Delay/1 -> SysID Kalman Filter/1
  strain/1 -> Unit Delay/1
  SysID Kalman Filter/1 -> Rate Transition/1
  Rate Transition/1 -> Bus Creator/1  "normal"
  Bus Creator/1 -> force_estimate/1

== system soft_finger_main/state_estimation/linear_regression ==
  strain : Inport
  Bus Creator : BusCreator  Inputs=1
  Rate Transition : RateTransition  InitialCondition=0;  OutPortSampleTime=1/cf;
  Unit Delay : UnitDelay  SampleTime=-1  HasFrameUpgradeWarning=on
  linear_regression : MATLAB Function  TreatAsAtomicUnit=on
  force_estimate : Outport
  wires:
  Unit Delay/1 -> linear_regression/1(Strain)
  strain/1 -> Unit Delay/1
  linear_regression/1(force) -> Rate Transition/1
  Rate Transition/1 -> Bus Creator/1  "normal"
  Bus Creator/1 -> force_estimate/1

== system soft_finger_main/state_estimation/off ==
  strain : Inport
  Bus Creator : BusCreator  Inputs=2
  Rate Transition : RateTransition  InitialCondition=0;  OutPortSampleTime=1/cf;
  Rate Transition1 : RateTransition  InitialCondition=0;  OutPortSampleTime=1/cf;
  Unit Delay : UnitDelay  SampleTime=-1  HasFrameUpgradeWarning=on
  Unit Delay1 : UnitDelay  SampleTime=-1  HasFrameUpgradeWarning=on
  friction_state_estimator : Subsystem
  normal_force_state_estimator : Subsystem
  force_estimate : Outport
  wires:
  Bus Creator/1 -> force_estimate/1
  Rate Transition/1 -> Bus Creator/1  "normal"
  strain/1 -> Unit Delay1/1, Unit Delay/1
  normal_force_state_estimator/1(Out1) -> Rate Transition/1
  Unit Delay/1 -> normal_force_state_estimator/1(In1)
  Unit Delay1/1 -> friction_state_estimator/1(In1)
  friction_state_estimator/1(Out1) -> Rate Transition1/1
  Rate Transition1/1 -> Bus Creator/2  "friction"

== system soft_finger_main/state_estimation/state_space_observer ==
  strain : Inport
  Bus Creator : BusCreator  Inputs=1
  Rate Transition : RateTransition  InitialCondition=0;  OutPortSampleTime=1/cf;
  State-Space : StateSpace  InitialCondition=0
  Unit Delay : UnitDelay  SampleTime=-1  HasFrameUpgradeWarning=on
  force_estimate : Outport
  wires:
  State-Space/1 -> Rate Transition/1
  strain/1 -> Unit Delay/1
  Unit Delay/1 -> State-Space/1
  Rate Transition/1 -> Bus Creator/1  "normal"
  Bus Creator/1 -> force_estimate/1

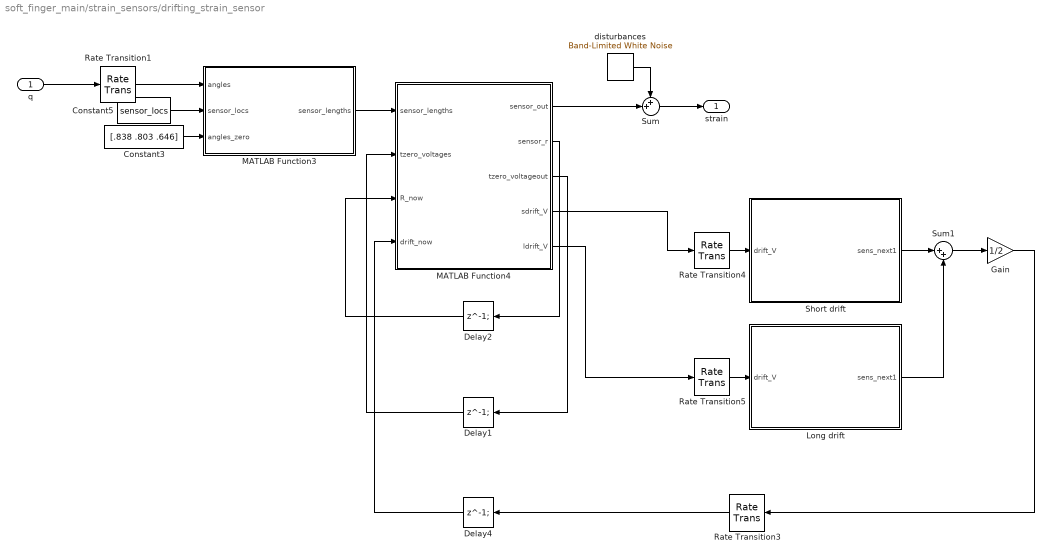
== system soft_finger_main/strain_sensors/drifting_strain_sensor ==
  q : Inport
  Constant3 : Constant  Value=[.838 .803 .646]
  Constant5 : Constant  Value=sensor_locs
  Delay1 : Delay  DelayLength=1;  InitialCondition=zeros(1,8)
  Delay2 : Delay  DelayLength=1;  InitialCondition=ones(1,8)*20000
  Delay4 : Delay  DelayLength=1;  InitialCondition=ones(1,8)*9600
  Gain : Gain  Gain=1/2
  Long drift : Subsystem
  MATLAB Function3 : MATLAB Function  TreatAsAtomicUnit=on
  MATLAB Function4 : MATLAB Function  TreatAsAtomicUnit=on
  Rate Transition1 : RateTransition  InitialCondition=0;  OutPortSampleTime=1/cf;
  Rate Transition3 : RateTransition  InitialCondition=ones(1,8)*5  OutPortSampleTime=1/cf;
  Rate Transition4 : RateTransition  InitialCondition=ones(1,8)*5  OutPortSampleTime=1/cf;
  Rate Transition5 : RateTransition  InitialCondition=ones(1,8)*5  OutPortSampleTime=1/cf;
  Short drift : Subsystem
  Sum : Sum  Inputs=++|
  Sum1 : Sum  Inputs=|++
  disturbances : simulink/Sources/Band-Limited White Noise  Cov=[0.000000013,0.000000013,0.000000013,0.000000013,0.000000013,0.000000013,0.000000013,0.000000013]  Ts=0.04  seed=[23341,23342,23343,23344,23345,23346,23347,23348]
  strain : Outport
  wires:
  Short drift/1(sens_next1) -> Sum1/1
  Long drift/1(sens_next1) -> Sum1/2
  MATLAB Function4/5(ldrift_V) -> Rate Transition5/1
  Constant3/1 -> MATLAB Function3/3(angles_zero)
  Gain/1 -> Rate Transition3/1
  Delay1/1 -> MATLAB Function4/2(tzero_voltages)
  Rate Transition1/1 -> MATLAB Function3/1(angles)
  MATLAB Function4/2(sensor_r) -> Delay2/1
  MATLAB Function4/3(tzero_voltageout) -> Delay1/1
  Rate Transition4/1 -> Short drift/1(drift_V)
  q/1 -> Rate Transition1/1
  Rate Transition3/1 -> Delay4/1
  Sum/1 -> strain/1
  Delay2/1 -> MATLAB Function4/3(R_now)
  Constant5/1 -> MATLAB Function3/2(sensor_locs)
  MATLAB Function3/1(sensor_lengths) -> MATLAB Function4/1(sensor_lengths)
  disturbances/1 -> Sum/1
  Delay4/1 -> MATLAB Function4/4(drift_now)
  MATLAB Function4/1(sensor_out) -> Sum/2
  Sum1/1 -> Gain/1
  Rate Transition5/1 -> Long drift/1(drift_V)
  MATLAB Function4/4(sdrift_V) -> Rate Transition4/1

== system soft_finger_main/strain_sensors/ssc_strain_sensor ==
  note: $F = \tau /R$
  tau : Inport
  Rate Transition1 : RateTransition  InitialCondition=0;  OutPortSampleTime=1/cf;
  Rate Transition2 : RateTransition  InitialCondition=0;  OutPortSampleTime=1/cf;
  Sum : Sum  Inputs=++|
  disturbances : simulink/Sources/Band-Limited White Noise  Cov=[0.000000013,0.000000013,0.000000013,0.000000013,0.000000013,0.000000013,0.000000013,0.000000013,0.000000013]/10  Ts=0.04  seed=[23341,23342,23343,23344,23345,23346,23347,23348,23349]
  sensor_model : Subsystem
  tau2surfaceForce : Gain  Gain=2/D/1e-3
  strain : Outport
  wires:
  tau/1 -> Rate Transition1/1
  disturbances/1 -> Sum/1
  sensor_model/1(strain) -> Sum/2
  Sum/1 -> Rate Transition2/1
  Rate Transition1/1 -> tau2surfaceForce/1
  Rate Transition2/1 -> strain/1
  tau2surfaceForce/1 -> sensor_model/1(force)

== system soft_finger_main/controller/contact_1D_controller/acceleration limiter ==
  pos_next : Inport
  Clock : Clock
  Delay : Delay  DelayLength=1  InitialCondition=[0,0]
  Demux : Demux  Outputs=2
  Derivative : Derivative  Commented=on
  Derivative1 : Derivative
  Integrator : Integrator  Commented=on  InitialConditionSource=external
  MATLAB Function : MATLAB Function  TreatAsAtomicUnit=on
  Mux : Mux  Inputs=2
  Rate Limiter : RateLimiter  RisingSlewLimit=6000  FallingSlewLimit=-6000
  Rate Limiter1 : RateLimiter  Commented=on  RisingSlewLimit=6000  FallingSlewLimit=-6000
  Subsystem : Subsystem  Commented=on
  zout : Outport
  wires:
  Derivative/1 -> Rate Limiter1/1
  Rate Limiter1/1 -> Integrator/1
  pos_next/1 -> Mux/1, MATLAB Function/1(zin), Derivative1/1
  Derivative1/1 -> Rate Limiter/1, MATLAB Function/2(zdot)
  Rate Limiter/1 -> MATLAB Function/3(zdotlimit)
  Clock/1 -> MATLAB Function/6(t), Mux/2
  Mux/1 -> Delay/1
  Delay/1 -> Demux/1
  Demux/2 -> MATLAB Function/5(tlast)
  Demux/1 -> MATLAB Function/4(zlast)
  MATLAB Function/1(zout) -> zout/1

== system soft_finger_main/controller/contact_2D_controller/acceleration limiter ==
  pos_next : Inport
  Clock : Clock
  Delay : Delay  DelayLength=1  InitialCondition=[0,0]
  Demux : Demux  Outputs=2
  Derivative : Derivative  Commented=on
  Derivative1 : Derivative
  Integrator : Integrator  Commented=on  InitialConditionSource=external
  MATLAB Function : MATLAB Function  TreatAsAtomicUnit=on
  Mux : Mux  Inputs=2
  Rate Limiter : RateLimiter  RisingSlewLimit=6000  FallingSlewLimit=-6000
  Rate Limiter1 : RateLimiter  Commented=on  RisingSlewLimit=6000  FallingSlewLimit=-6000
  Subsystem : Subsystem  Commented=on
  zout : Outport
  wires:
  MATLAB Function/1(zout) -> zout/1
  Demux/1 -> MATLAB Function/4(zlast)
  Demux/2 -> MATLAB Function/5(tlast)
  Delay/1 -> Demux/1
  Mux/1 -> Delay/1
  Clock/1 -> Mux/2, MATLAB Function/6(t)
  Rate Limiter/1 -> MATLAB Function/3(zdotlimit)
  Derivative1/1 -> MATLAB Function/2(zdot), Rate Limiter/1
  pos_next/1 -> Derivative1/1, MATLAB Function/1(zin), Mux/1
  Rate Limiter1/1 -> Integrator/1
  Derivative/1 -> Rate Limiter1/1

== system soft_finger_main/controller/random_walker_z/acceleration limiter ==
  pos_next : Inport
  Clock : Clock
  Delay : Delay  DelayLength=1  InitialCondition=[0,0]
  Demux : Demux  Outputs=2
  Derivative1 : Derivative
  MATLAB Function : MATLAB Function  TreatAsAtomicUnit=on
  Mux : Mux  Inputs=2
  Rate Limiter : RateLimiter  RisingSlewLimit=6000  FallingSlewLimit=-6000
  zout : Outport
  wires:
  pos_next/1 -> Derivative1/1, MATLAB Function/1(zin), Mux/1
  Derivative1/1 -> Rate Limiter/1, MATLAB Function/2(zdot)
  Rate Limiter/1 -> MATLAB Function/3(zdotlimit)
  Clock/1 -> MATLAB Function/6(t), Mux/2
  Mux/1 -> Delay/1
  Delay/1 -> Demux/1
  Demux/2 -> MATLAB Function/5(tlast)
  Demux/1 -> MATLAB Function/4(zlast)
  MATLAB Function/1(zout) -> zout/1
